simulink model "wing_example_sim"  (R2018b)
settings: Solver=FixedStepAuto  StartTime=0.0  StopTime=10  FixedStep=0.01  RelTol=1e-3
values from neighbouring files (symbols this model uses):
  wing = wingSetState(wing, alpha, beta, V, omega,      actuators_pos, actuators_rate, xyz_cg, 'atmosphere', isAtmosphere(h),      'V_Wb', zeros( 3, wing.n_panel ), 'V_Wb_dt', zeros( 3, wing.n_panel ) )    [wing_example.m]    (also in wing_example_Arkbird.m = wingSetState(wing, alpha, beta, V, omega,      actuators_pos; wing_example_geometry_from_CPACS.m = wingSetState(wing, alpha, beta, V, omega,      [ actuatorsLe; wing_example_polar.m = wingCreate('wing_params_Arkbird_simple',50); wing_example_sim_init.m = wingCreate('wing_params_Arkbird_simple',30))
libraries: atmosphere_lib x1, axes_transformation_lib x1, vlm_wing_lib x1
settings Model: Creator=Yannic  LastModifiedBy=yannic

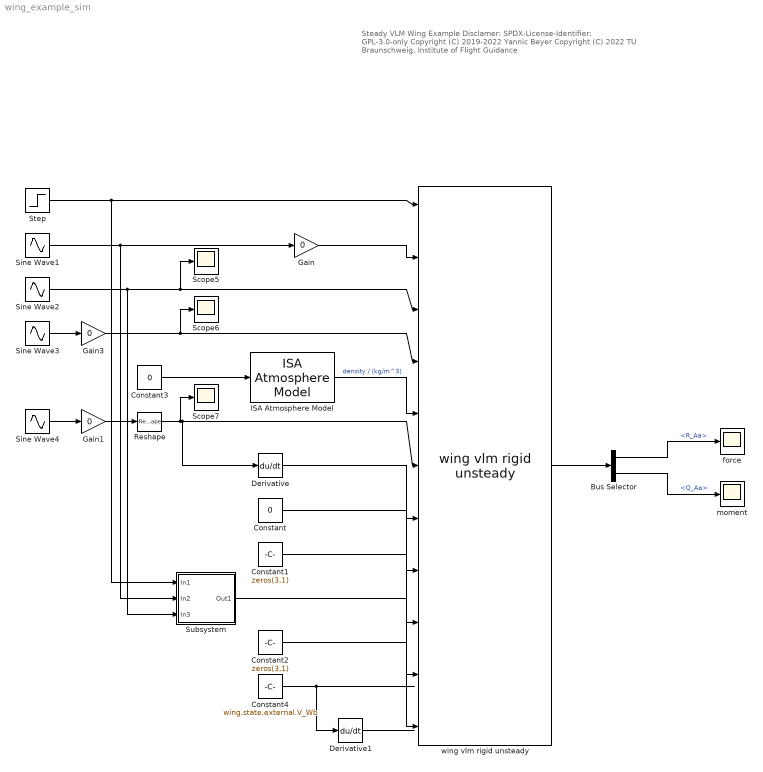
== system wing_example_sim ==
  note: Steady VLM Wing Example
      |
      | Disclamer:
      | SPDX-License-Identifier: GPL-3.0-only
      |
      | Copyright (C) 2019-2022 Yannic Beyer
      | Copyright (C) 2022 TU Braunschweig, Institute of Flight Guidance
  Bus Selector : BusSelector  OutputSignals=R_Aa,Q_Aa
  Constant : Constant  Value=0
  Constant1 : Constant  Value=zeros(3,1)  VectorParams1D=off
  Constant2 : Constant  Value=zeros(3,1)  VectorParams1D=off
  Constant3 : Constant  Value=0
  Constant4 : Constant  Value=wing.state.external.V_Wb
  Derivative : Derivative
  Derivative1 : Derivative
  Gain : Gain  Gain=0
  Gain1 : Gain  Gain=0
  Gain3 : Gain  Gain=0
  ISA Atmosphere Model : atmosphere_lib/ISA Atmosphere Model
      settings: SourceProductName=LADAC
  Reshape : Reshape  OutputDimensionality=Row vector (2-D)
  Scope5 : Scope
  Scope6 : Scope
  Scope7 : Scope
  Sine Wave1 : Sin  Amplitude=0.05  Frequency=0.3  SampleTime=0
  Sine Wave2 : Sin  Amplitude=3  Bias=100  Frequency=0.22  SampleTime=0
  Sine Wave3 : Sin  Amplitude=[0.1;0.1;0.1]  Frequency=[0.9;0.8;0.7]  SampleTime=0
  Sine Wave4 : Sin  Amplitude=[0.1;0.1]  Frequency=[0.9;0.8]*2.1  SampleTime=0
  Step : Step  Time=0.01  After=0.1  SampleTime=0
  Subsystem : Subsystem
  force : Scope
  moment : Scope
  wing vlm rigid unsteady : vlm_wing_lib/wing vlm rigid unsteady  wing_struct=wing  wing_state_bus=wing_state_bus  unst_aero_state_init=0  dyn_stall_state_init=0  unst_flap_state_init=0  unst_act2_state_init=0  tau_v_init=0  alpha_ind_init=0
      settings: SourceProductName=LADAC
  wires:
  Constant3/1 -> ISA Atmosphere Model/1
  Sine Wave4/1 -> Gain1/1
  Constant1/1 -> wing vlm rigid unsteady/9
  Sine Wave2/1 -> wing vlm rigid unsteady/3, Scope5/1, Subsystem/3(In3)
  Bus Selector/2 -> moment/1  "<Q_Aa>"
  Derivative/1 -> wing vlm rigid unsteady/7
  Bus Selector/1 -> force/1  "<R_Aa>"
  Reshape/1 -> Scope7/1, wing vlm rigid unsteady/6, Derivative/1
  wing vlm rigid unsteady/1 -> Bus Selector/1
  Gain3/1 -> wing vlm rigid unsteady/4, Scope6/1
  ISA Atmosphere Model/1 -> wing vlm rigid unsteady/5  "density / (kg/m^3)"
  Gain1/1 -> Reshape/1
  Constant/1 -> wing vlm rigid unsteady/8
  Sine Wave1/1 -> Gain/1, Subsystem/2(In2)
  Step/1 -> Subsystem/1(In1), wing vlm rigid unsteady/1
  Gain/1 -> wing vlm rigid unsteady/2
  Sine Wave3/1 -> Gain3/1
  Constant4/1 -> Derivative1/1
  Derivative1/1 -> ?
  Constant2/1 -> wing vlm rigid unsteady/11
  Subsystem/1(Out1) -> wing vlm rigid unsteady/10

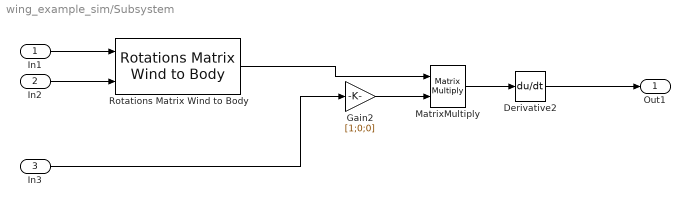
== system wing_example_sim/Subsystem ==
  In1 : Inport
  In2 : Inport  Port=2
  In3 : Inport  Port=3
  Derivative2 : Derivative
  Gain2 : Gain  Gain=[1;0;0]
  MatrixMultiply : Product  Multiplication=Matrix(*)
  Rotations Matrix Wind to Body : axes_transformation_lib/Rotations Matrix Wind to Body  SystemSampleTime=-1
      settings: SourceProductName=LADAC
  Out1 : Outport
  wires:
  Gain2/1 -> MatrixMultiply/2
  Rotations Matrix Wind to Body/1 -> MatrixMultiply/1
  MatrixMultiply/1 -> Derivative2/1
  In1/1 -> Rotations Matrix Wind to Body/1
  Derivative2/1 -> Out1/1
  In3/1 -> Gain2/1
  In2/1 -> Rotations Matrix Wind to Body/2
